simulink model "vidvig_example"  (R2021a)
settings: Solver=VariableStepAuto  StartTime=0.0  StopTime=10  RelTol=1e-3
values from neighbouring files (symbols this model uses):
  alpha_1M = 0.9*Xmax1    (= 27)    [NASTROYKI.m]    (also in NASTROYKI_STAB.m; NASTROYKI_VSEGO.m)
  DtR = pi/180    (= 0.0174532925199)    [NASTROYKI.m]    (also in NASTROYKI_STAB.m; NASTROYKI_VSEGO.m)
  h_1M = 0.2*alpha_1M    (= 5.4)    [NASTROYKI.m]    (also in NASTROYKI_STAB.m; NASTROYKI_VSEGO.m)
  J1K = 6937    [NASTROYKI.m]    (also in NASTROYKI_STAB.m; NASTROYKI_VSEGO.m)
  J1Knew = 10000    [NASTROYKI_VSEGO.m]
  J1M = 2    [NASTROYKI.m]    (also in NASTROYKI_STAB.m; NASTROYKI_VSEGO.m)
  k_1M = h_1M/(2*yZV)    (= 2.7)    [NASTROYKI.m]    (also in NASTROYKI_STAB.m; NASTROYKI_VSEGO.m)
  M1B = 1e-5    (= 1e-05)    [NASTROYKI.m]    (also in NASTROYKI_STAB.m; NASTROYKI_VSEGO.m)
  M1U = 20    [KUBSAT_NASTR.m]    (also in NASTROYKI.m = 10.64; NASTROYKI_VSEGO.m)
  RtD = 1/DtR    (= 57.2957795131)    [NASTROYKI.m]    (also in NASTROYKI_STAB.m; NASTROYKI_VSEGO.m)
  x_0_1M = xZV    (= 30)    [NASTROYKI.m]    (also in NASTROYKI_STAB.m; NASTROYKI_VSEGO.m)
  y_0_1M = yZV    (= 1)    [NASTROYKI.m]    (also in NASTROYKI_STAB.m; NASTROYKI_VSEGO.m)
libraries: shared6dof x1, aerolibanim x1
settings Model: Creator=vanya  LastModifiedBy=vanya

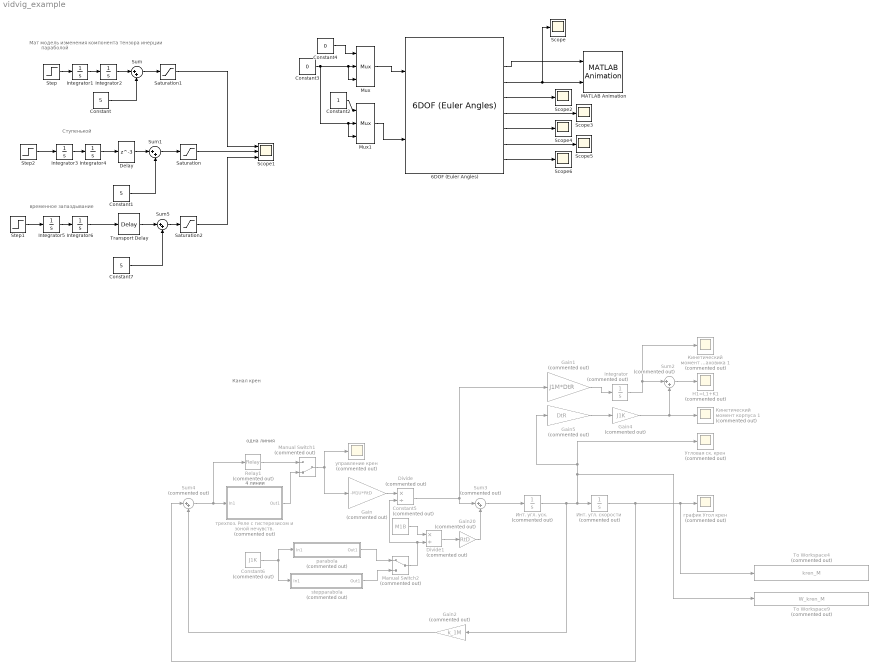
== system vidvig_example ==
  note: временное запаздывание
  note: Мат модель изменения компонента тензора инерции
  note: 4 линии
  note: одна линия
  note: параболой
  note: Ступенькой
  note: Канал
      | крен
  " Кинетический момент корпуса 1" : Scope  Commented=on
  6DOF (Euler Angles) : shared6dof/6DOF (Euler Angles)  units=Metric (MKS)  mtype=Fixed  rep=Euler Angles  xme_0=[0 0 0]  Vm_0=[0 0 0]  eul_0=[0 0 0]  pm_0=[0 0 0]  mass_0=1.0  mass_e=0.5  mass_f=2.0  inertia=I  inertia_e=eye(3)  inertia_f=2*eye(3)  k_quat=1.0  vre_flag=on  abi_flag=off  aMode=0  xme_statename=''  Vm_statename=''  eul_statename=''  quat_statename=''  pm_statename=''  mass_statename=''
      settings: SourceProductBaseCode=AE,PW,DR,MT,UV,VE
  Constant : Constant  Value=5
  Constant1 : Constant  Value=5
  Constant2 : Constant
  Constant3 : Constant  Value=0
  Constant4 : Constant  Value=0
  Constant5 : Constant  Commented=on  Value=M1B
  Constant6 : Constant  Commented=on  Value=J1K
  Constant7 : Constant  Value=5
  Delay : Delay  DelayLength=3  InputProcessing=Columns as channels (frame based)
  Divide : Product  Commented=on  Inputs=*/
  Divide1 : Product  Commented=on  Inputs=*/
  Gain : Gain  Commented=on  Gain=-M1U*RtD
  Gain1 : Gain  Commented=on  Gain=J1M*DtR
  Gain2 : Gain  Commented=on  Gain=k_1M
  Gain20 : Gain  Commented=on  Gain=RtD
  Gain4 : Gain  Commented=on  Gain=J1K
  Gain5 : Gain  Commented=on  Gain=DtR
  H1=L1+K1 : Scope  Commented=on
  Integrator : Integrator  Commented=on
  Integrator{1..6} (6 alike) : Integrator
  MATLAB Animation : aerolibanim/MATLAB Animation  Tag=Matlab Animation 6 DOF  Vehicles=1  Geometries='astredwedge.mat'  BoundingBoxCoordinates=[-50,50,-50,50,-50,50]  CameraOffset=[150,150,-150]  CameraViewAngle=2  SampleTime=0.2  FigurePosition=[732,165,717,452]
      settings: SourceProductBaseCode=AE
  Manual Switch1 : ManualSwitch  Commented=on  CurrentSetting=0
  Manual Switch2 : ManualSwitch  Commented=on
  Mux : Mux  Inputs=3
  Mux1 : Mux  Inputs=3
  Relay1 : Relay  Commented=on  OnSwitchValue=0  OffSwitchValue=0  OffOutputValue=-1
  Saturation : Saturate  UpperLimit=10  LowerLimit=0
  Saturation1 : Saturate  UpperLimit=10  LowerLimit=0
  Saturation2 : Saturate  UpperLimit=10  LowerLimit=0
  Scope{,2..6} (6 alike) : Scope
  Scope1 : Scope  NumInputPorts=3
  Step : Step  Time=5  SampleTime=0
  Step1 : Step  Time=5  SampleTime=0
  Step2 : Step  Time=5  SampleTime=0
  Sum : Sum  Inputs=|++
  Sum1 : Sum  Inputs=|++
  Sum2 : Sum  Commented=on  Inputs=|++
  Sum3 : Sum  Commented=on  Inputs=|++
  Sum4 : Sum  Commented=on  Inputs=|++
  Sum5 : Sum  Inputs=|++
  To Workspace4 : ToWorkspace  Commented=on  VariableName=kren_M  SampleTime=-1
      settings: Save2DSignal=2-D array (concatenate along first dimension)
  To Workspace9 : ToWorkspace  Commented=on  VariableName=W_kren_M  SampleTime=-1
      settings: Save2DSignal=2-D array (concatenate along first dimension)
  Transport Delay : TransportDelay
  parabola : Subsystem  Commented=on
  stepparabola : Subsystem  Commented=on
  Инт. угл. скорости : Integrator  Commented=on  InitialCondition=x_0_1M
  Инт. угл. уск. : Integrator  Commented=on  InitialCondition=y_0_1M
  Кинетический момент маховика 1 : Scope  Commented=on
  Угловая ск. крен : Scope  Commented=on
  график Угол крен : Scope  Commented=on
  трехпоз. Реле с гистерезисом и зоной нечувств. : Subsystem  Commented=on
  управление крен : Scope  Commented=on
  wires:
  Saturation/1 -> Scope1/2
  Step2/1 -> Integrator3/1
  Sum1/1 -> Saturation/1
  Saturation1/1 -> Scope1/1
  Step/1 -> Integrator1/1
  Sum/1 -> Saturation1/1
  Constant/1 -> Sum/2
  Constant1/1 -> Sum1/2
  Delay/1 -> Sum1/1
  Integrator4/1 -> Delay/1
  Mux/1 -> 6DOF (Euler Angles)/1
  Mux1/1 -> 6DOF (Euler Angles)/2
  Constant2/1 -> Mux1/1
  Constant3/1 -> Mux/2, Mux/3, Mux1/3, Mux1/2
  6DOF (Euler Angles)/3 -> Scope/1, MATLAB Animation/2
  6DOF (Euler Angles)/2 -> MATLAB Animation/1
  Constant4/1 -> Mux/1
  6DOF (Euler Angles)/4 -> Scope2/1
  6DOF (Euler Angles)/5 -> Scope3/1
  6DOF (Euler Angles)/6 -> Scope4/1
  6DOF (Euler Angles)/7 -> Scope5/1
  6DOF (Euler Angles)/8 -> Scope6/1
  Gain1/1 -> Integrator/1
  Manual Switch1/1 -> Gain/1, управление крен/1
  Divide/1 -> Sum3/1, Gain1/1
  Relay1/1 -> Manual Switch1/1
  трехпоз. Реле с гистерезисом и зоной нечувств./1(Out1) -> Manual Switch1/2
  Divide1/1 -> Gain20/1
  Инт. угл. уск./1 -> Gain2/1, To Workspace9/1, Gain5/1, Угловая ск. крен/1, Инт. угл. скорости/1
  Gain4/1 -> " Кинетический момент корпуса 1"/1, Sum2/2
  Gain20/1 -> Sum3/2
  Gain5/1 -> Gain4/1
  Инт. угл. скорости/1 -> график Угол крен/1, To Workspace4/1, Sum4/1
  Integrator/1 -> Кинетический момент маховика 1/1, Sum2/1
  Sum4/1 -> трехпоз. Реле с гистерезисом и зоной нечувств./1(In1), Relay1/1
  Sum3/1 -> Инт. угл. уск./1
  Gain2/1 -> Sum4/2
  Sum2/1 -> H1=L1+K1/1
  Constant5/1 -> Divide1/1
  Manual Switch2/1 -> Divide/2, Divide1/2
  stepparabola/1(Out1) -> Manual Switch2/2
  parabola/1(Out1) -> Manual Switch2/1
  Gain/1 -> Divide/1
  Constant6/1 -> stepparabola/1(In1), parabola/1(In1)
  Step1/1 -> Integrator5/1
  Saturation2/1 -> Scope1/3
  Integrator6/1 -> Transport Delay/1
  Transport Delay/1 -> Sum5/1
  Constant7/1 -> Sum5/2
  Sum5/1 -> Saturation2/1
  Integrator1/1 -> Integrator2/1
  Integrator2/1 -> Sum/1
  Integrator3/1 -> Integrator4/1
  Integrator5/1 -> Integrator6/1

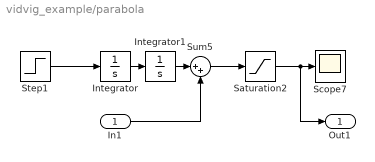
== system vidvig_example/parabola ==
  In1 : Inport
  Integrator : Integrator
  Integrator1 : Integrator
  Saturation2 : Saturate  UpperLimit=J1Knew  LowerLimit=0
  Scope7 : Scope
  Step1 : Step  Time=5  SampleTime=0
  Sum5 : Sum  Inputs=|++
  Out1 : Outport
  wires:
  Saturation2/1 -> Out1/1, Scope7/1
  Sum5/1 -> Saturation2/1
  Step1/1 -> Integrator/1
  In1/1 -> Sum5/2
  Integrator/1 -> Integrator1/1
  Integrator1/1 -> Sum5/1

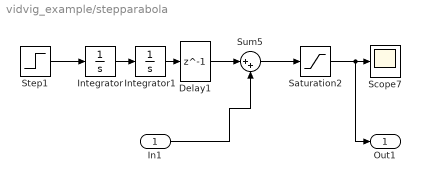
== system vidvig_example/stepparabola ==
  In1 : Inport
  Delay1 : Delay  DelayLength=1  InputProcessing=Columns as channels (frame based)
  Integrator : Integrator
  Integrator1 : Integrator
  Saturation2 : Saturate  UpperLimit=J1Knew  LowerLimit=0
  Scope7 : Scope
  Step1 : Step  Time=5  SampleTime=0
  Sum5 : Sum  Inputs=|++
  Out1 : Outport
  wires:
  Sum5/1 -> Saturation2/1
  Saturation2/1 -> Out1/1, Scope7/1
  In1/1 -> Sum5/2
  Step1/1 -> Integrator/1
  Delay1/1 -> Sum5/1
  Integrator/1 -> Integrator1/1
  Integrator1/1 -> Delay1/1

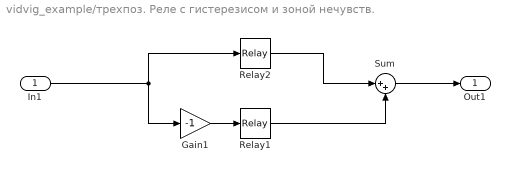
== system vidvig_example/трехпоз. Реле с гистерезисом и зоной нечувств. ==
  In1 : Inport
  Gain1 : Gain  Gain=-1
  Relay1 : Relay  OnSwitchValue=alpha_1M  OffSwitchValue=alpha_1M-h_1M  OnOutputValue=-1
  Relay2 : Relay  OnSwitchValue=alpha_1M  OffSwitchValue=alpha_1M-h_1M
  Sum : Sum  Inputs=|++
  Out1 : Outport
  wires:
  Gain1/1 -> Relay1/1
  In1/1 -> Gain1/1, Relay2/1
  Sum/1 -> Out1/1
  Relay1/1 -> Sum/2
  Relay2/1 -> Sum/1
